simulink model "Smart_City_QCar2_self_driving_stack"  (R2024b)
settings: Solver=ode1  StartTime=0.0  StopTime=inf  FixedStep=Controller_Sample_Time  RelTol=1e-3  EnableMultiTasking=on
values from neighbouring files (symbols this model uses):
  angles_qcar2 = angles_new_qcar2(2: length (angles_new_qcar2), width (angles_new_qcar2)-5)    [Setup_QCar1and2_params.m]
  Audio_Sample_Time = 0.3    [Setup_QCar1and2_params.m]
  cal_pos = [0, 0, 0]    [Setup_QCar1and2_params.m]
  cameraStepSize = 3e-2    (= 0.03)    [Setup_QCar1and2_params.m]
  Cobra_Start = [0 0 0 0 0 0 0 0 0 0 0 0 ... (192000 elements, 192000x1)]    [QCar_Sounds.mat]
  Controller_Sample_Time = CSI_Sample_Time/10    (= 0.00166666666667)    [Setup_QCar1and2_params.m]
  CSI_Sample_Time = 1/60    (= 0.0166666666667)    [Setup_QCar1and2_params.m]
  engine = [0.455749511719 0.619506835938 0.612854003906 0.499603271484 0.347473144531 0.278045654297 0.304656982422 0.258544921875 0.100128173828 0.0902099609375 0.341461181641 0.515716552734 ... (88200 elements, 44100x2)]    [QCar_Sounds.mat]
  GyroKF_P0 = eye(2)    [Setup_QCar1and2_params.m]
  GyroKF_Q = diag([0.01, 0.001])    [Setup_QCar1and2_params.m]
  GyroKF_R = 0.01    [Setup_QCar1and2_params.m]
  GyroKF_X0 = [0;0]    [Setup_QCar1and2_params.m]
  honk = [0.01708984375 0.0179443359375 0.018798828125 0.019775390625 0.0209655761719 0.0218505859375 0.0221557617188 0.0223693847656 0.022705078125 0.023681640625 0.0252075195312 0.0257263183594 ... (43568 elements, 21784x2)]    [QCar_Sounds.mat]
  ImageDisplay_Sample_Time = CSI_Sample_Time*6    (= 0.1)    [Setup_QCar1and2_params.m]
  Initialization_Time = 5    [Setup_QCar1and2_params.m]
  LiDAR_Sample_Time = CSI_Sample_Time*3    (= 0.05)    [Setup_QCar1and2_params.m]
  map_mask = [1 1 1 0 0 1 0]    [Setup_QCar1and2_params.m]
  NN_Sample_Time = RealSense_Sample_Time*1    (= 0.0333333333333)    [Setup_QCar1and2_params.m]
  path_x = [0.826 0.836 0.846 0.856 0.866 0.876 0.886 0.896 0.906 0.916 0.926 0.936 ... (740 elements, 740x1)]    [SDCS_Paths_7.mat]
  path_x2 = [-0.614 -0.604 -0.594 -0.584 -0.574 -0.564 -0.554 -0.544 -0.534 -0.524 -0.514 -0.504 ... (1090 elements, 1090x1)]    [SDCS_Paths_7.mat]
  path_x3 = [-0.614 -0.603821428571 -0.593642857143 -0.583464285714 -0.573285714286 -0.563107142857 -0.552928571429 -0.54275 -0.532571428571 -0.522392857143 -0.512214285714 -0.502035714286 ... (714 elements, 714x1)]    [SDCS_Paths_7.mat]
  path_x4 = [-0.614 -0.604 -0.594 -0.584 -0.574 -0.564 -0.554 -0.544 -0.534 -0.524 -0.514 -0.504 ... (1761 elements, 1761x1)]    [SDCS_Paths_7.mat]
  path_x5 = [1.436 1.42588571429 1.41577142857 1.40565714286 1.39554285714 1.38542857143 1.37531428571 1.3652 1.35508571429 1.34497142857 1.33485714286 1.32474285714 ... (574 elements, 574x1)]    [SDCS_Paths_7.mat]
  path_x6 = [1.436 1.42588571429 1.41577142857 1.40565714286 1.39554285714 1.38542857143 1.37531428571 1.3652 1.35508571429 1.34497142857 1.33485714286 1.32474285714 ... (1288 elements, 1288x1)]    [SDCS_Paths_7.mat]
  path_x7 = [-1.5778487585 -1.56959877056 -1.56127865467 -1.55288878259 -1.54442952915 -1.53590127231 -1.52730439309 -1.51863927561 -1.50990630701 -1.50110587746 -1.49223838016 -1.4833042113 ... (2260 elements, 2260x1)]    [SDCS_Paths_7.mat]
  path_y = [-1.0887 -1.0887 -1.0887 -1.0887 -1.0887 -1.0887 -1.0887 -1.0887 -1.0887 -1.0887 -1.0887 -1.0887 ... (740 elements, 740x1)]    [SDCS_Paths_7.mat]
  path_y2 = [-1.0887 -1.0887 -1.0887 -1.0887 -1.0887 -1.0887 -1.0887 -1.0887 -1.0887 -1.0887 -1.0887 -1.0887 ... (1090 elements, 1090x1)]    [SDCS_Paths_7.mat]
  path_y3 = [-1.0887 -1.0887 -1.0887 -1.0887 -1.0887 -1.0887 -1.0887 -1.0887 -1.0887 -1.0887 -1.0887 -1.0887 ... (714 elements, 714x1)]    [SDCS_Paths_7.mat]
  path_y4 = [-1.0887 -1.0887 -1.0887 -1.0887 -1.0887 -1.0887 -1.0887 -1.0887 -1.0887 -1.0887 -1.0887 -1.0887 ... (1761 elements, 1761x1)]    [SDCS_Paths_7.mat]
  path_y5 = [-0.8157 -0.8157 -0.8157 -0.8157 -0.8157 -0.8157 -0.8157 -0.8157 -0.8157 -0.8157 -0.8157 -0.8157 ... (574 elements, 574x1)]    [SDCS_Paths_7.mat]
  path_y6 = [-0.8157 -0.8157 -0.8157 -0.8157 -0.8157 -0.8157 -0.8157 -0.8157 -0.8157 -0.8157 -0.8157 -0.8157 ... (1288 elements, 1288x1)]    [SDCS_Paths_7.mat]
  path_y7 = [-0.614490295955 -0.61974988896 -0.624981792226 -0.630185771997 -0.635361595765 -0.640509032279 -0.645627851559 -0.6507178249 -0.655778724888 -0.660810325409 -0.665812401655 -0.670784730139 ... (2260 elements, 2260x1)]    [SDCS_Paths_7.mat]
  put_me_down = [0 0 0 0 0 0 0 0 0 0 0 0 ... (335870 elements, 167935x2)]    [QCar_Sounds.mat]
  qcar2_lidar_to_map_rotation = 0    [Setup_QCar1and2_params.m]
  QCarEKF_L = 0.24    [Setup_QCar1and2_params.m]
  QCarEKF_P0 = eye(3)    [Setup_QCar1and2_params.m]
  QCarEKF_Q = diag([0.00001, 0.00001, 0.00001])    [Setup_QCar1and2_params.m]
  QCarEKF_R_combined = diag([0.1, 0.1, 0.01])    [Setup_QCar1and2_params.m]
  QCarEKF_R_heading = diag(0.1)    [Setup_QCar1and2_params.m]
  QcarKF_X0 = [0; 0; 0]    [Setup_QCar1and2_params.m]
  range_qcar2 = distance_new_qcar2(2: length (distance_new_qcar2), width (distance_new_qcar2)-5)    [Setup_QCar1and2_params.m]
  RealSense_Sample_Time = CSI_Sample_Time*2    (= 0.0333333333333)    [Setup_QCar1and2_params.m]
  truck_start = [0.00137329101562 0.00115966796875 0.0006103515625 0.000762939453125 0.00115966796875 0.00198364257812 0.00115966796875 0.000762939453125 0.00137329101562 0.00115966796875 0.00115966796875 0.000762939453125 ... (60000 elements, 60000x1)]    [QCar_Sounds.mat]
undefined symbols (not defined in the file or in its folder): DiscIntNeverNeededParam, gcbh, height, HIL, Joystick_Sample_Time, JPEG, left, Point, qc_get_step_size, top, video_display_show, width
libraries: quarc_library x65, simulink_extras x12, simulink x8
(part 4 of 5)

== system Smart_City_QCar2_self_driving_stack/QCar 2/QCar Control/QCar I//O/Audio ==
  Honk : Inport
  Arm : Inport  Port=2
  put_me_down : Inport  Port=3
  Volume : Inport  Port=4
  Car Horn1 : Constant  Value=[honk; honk]  VectorParams1D=off  OutDataTypeStr=single  SampleTime=Audio_Sample_Time
  Car Speaker1 : Subsystem
  Data Type Conversion : DataTypeConversion  OutDataTypeStr=single  SaturateOnIntegerOverflow=off  RndMeth=Floor
  From3 : From  Commented=on  GotoTag=Volume
  Old Car Engine2 : Constant  Commented=on  Value=engine  VectorParams1D=off  OutDataTypeStr=single  SampleTime=Audio_Sample_Time
  Old Car Engine3 : Constant  Commented=on  Value=truck_start  VectorParams1D=off  OutDataTypeStr=single  SampleTime=1
  Old Car Engine4 : Constant  Value=Cobra_Start  VectorParams1D=off  OutDataTypeStr=single  SampleTime=Audio_Sample_Time
  Old Car Engine5 : Constant  Value=put_me_down  VectorParams1D=off  OutDataTypeStr=single  SampleTime=Audio_Sample_Time
  Product11 : Product
  Product5 : Product
  Product8 : Product  Commented=on
  Rate Transition{,1,4..5} (4 alike) : RateTransition
  Rate Transition3 : RateTransition  Commented=on
  Subsystem2 : Subsystem  Commented=on
  Subsystem3 : Subsystem  Commented=on
  Subsystem4 : Subsystem
  Subsystem5 : Subsystem
  Volume4 : Gain  Commented=on  Gain=1/30  ParamDataTypeStr=double  OutDataTypeStr=single
  Volume5 : Gain  Gain=5/30  ParamDataTypeStr=double  OutDataTypeStr=single
  Volume7 : Gain  Commented=on  Gain=30/30  ParamDataTypeStr=double  OutDataTypeStr=single
  Volume8 : Gain  Gain=30/30*1  ParamDataTypeStr=double  OutDataTypeStr=single
  Volume9 : Gain  Gain=20/30  ParamDataTypeStr=double  OutDataTypeStr=single
  wires:
  Honk/1 -> Rate Transition/1
  Arm/1 -> Rate Transition1/1
  Rate Transition1/1 -> Subsystem2/Enable, Product5/2, Subsystem4/Trigger
  Old Car Engine2/1 -> Volume4/1
  Rate Transition/1 -> Product5/1
  Car Horn1/1 -> Volume5/1
  Old Car Engine3/1 -> Volume7/1
  Volume7/1 -> Subsystem3/1(In1)
  Product5/1 -> Car Speaker1/Enable
  Old Car Engine5/1 -> Volume9/1
  Volume9/1 -> Subsystem5/1(In1)
  Rate Transition4/1 -> Subsystem5/Enable
  put_me_down/1 -> Rate Transition4/1
  Volume/1 -> Rate Transition5/1
  Rate Transition5/1 -> Data Type Conversion/1
  From3/1 -> Product8/1
  Product8/1 -> Subsystem2/1(In1)
  Volume4/1 -> Product8/2
  [Volume] -> Product11/1
  Product11/1 -> Car Speaker1/1(chs)
  Volume5/1 -> Product11/2
  Data Type Conversion/1 -> [Volume]
  Old Car Engine4/1 -> Volume8/1
  Volume8/1 -> Subsystem4/1(In1)

== system Smart_City_QCar2_self_driving_stack/QCar 2/QCar Control/QCar I//O/Greater Than Threshold ==
  Signal : Inport
  Threshold : Inport  Port=2
  Duration : Inport  Port=3
  Data Type Conversion : DataTypeConversion  SaturateOnIntegerOverflow=off  RndMeth=Floor
  Discrete-Time Integrator : DiscreteIntegrator  Priority=1  ExternalReset=level  SampleTime=qc_get_step_size  ICPrevOutput=DiscIntNeverNeededParam  ICPrevScaledInput=DiscIntNeverNeededParam
  Logical Operator : Logic  Operator=NOT  AllPortsSameDT=off  OutDataTypeStr=boolean
  Relational Operator : RelationalOperator  InputSameDT=off
  Relational Operator1 : RelationalOperator  InputSameDT=off
  elapsed : Outport  VectorParamsAs1DForOutWhenUnconnected=off
  time : Outport  Port=2  VectorParamsAs1DForOutWhenUnconnected=off
  wires:
  Relational Operator1/1 -> elapsed/1
  Duration/1 -> Relational Operator1/2
  Discrete-Time Integrator/1 -> time/1, Relational Operator1/1
  Logical Operator/1 -> Discrete-Time Integrator/2
  Relational Operator/1 -> Logical Operator/1, Data Type Conversion/1
  Threshold/1 -> Relational Operator/2
  Signal/1 -> Relational Operator/1
  Data Type Conversion/1 -> Discrete-Time Integrator/1

== system Smart_City_QCar2_self_driving_stack/QCar 2/QCar Control/QCar I//O/LEDs ==
  note: Headlights, Brakes, Left, Right
  Throttle : Inport
  Steering : Inport  Port=2
  Speed : Inport  Port=3
  Hazzard : Inport  Port=4
  AND : Logic  IconShape=distinctive  AllPortsSameDT=off  OutDataTypeStr=boolean
  Constant : Constant  OutDataTypeStr=boolean
  Constant1 : Constant  Value=10
  Constant{2,4,6..7} (4 alike) : Constant  Value=.1
  Constant3 : Constant  Value=0
  Constant5 : Constant  Value=0
  Constant8 : Constant  Value=eps
  Demux : Demux
  Gain : Gain  Gain=-1
  Gain1 : Gain  Gain=-1
  Greater Than Threshold : Subsystem
  Greater Than Threshold1 : Subsystem
  Less Than Threshold : Subsystem
  Less Than Threshold1 : Subsystem
  Less Than Threshold2 : Subsystem
  Less Than Threshold3 : Subsystem
  Mux : Mux
  OR : Logic  Operator=OR  IconShape=distinctive  AllPortsSameDT=off  OutDataTypeStr=boolean
  Radians to Degrees : simulink_extras/Transformations/Radians to Degrees
  indicatorAndLamps : Subsystem
  LEDs : Outport
  wires:
  indicatorAndLamps/1(LEDs) -> LEDs/1
  Steering/1 -> Radians to Degrees/1
  Radians to Degrees/1 -> Less Than Threshold/1(Signal), Greater Than Threshold/1(Signal)
  Constant1/1 -> Gain/1, Greater Than Threshold/2(Threshold)
  Constant2/1 -> Less Than Threshold/3(Duration), Greater Than Threshold/3(Duration)
  Greater Than Threshold/1(elapsed) -> Mux/3
  Gain/1 -> Less Than Threshold/2(Threshold)
  Less Than Threshold/1(elapsed) -> Mux/4
  Speed/1 -> Less Than Threshold3/1(Signal), Greater Than Threshold1/1(Signal), Less Than Threshold1/1(Signal)
  Constant3/1 -> Less Than Threshold1/2(Threshold)
  Constant4/1 -> Less Than Threshold1/3(Duration)
  Less Than Threshold1/1(elapsed) -> indicatorAndLamps/5(reverse)
  Throttle/1 -> Less Than Threshold2/1(Signal)
  Constant5/1 -> Less Than Threshold2/2(Threshold)
  Constant6/1 -> Less Than Threshold2/3(Duration)
  Hazzard/1 -> indicatorAndLamps/6(hazard)
  Less Than Threshold2/1(elapsed) -> OR/1
  Constant7/1 -> Less Than Threshold3/3(Duration), Greater Than Threshold1/3(Duration)
  Constant8/1 -> Gain1/1, Less Than Threshold3/2(Threshold)
  Less Than Threshold3/1(elapsed) -> AND/1
  Greater Than Threshold1/1(elapsed) -> AND/2
  AND/1 -> OR/2
  Gain1/1 -> Greater Than Threshold1/2(Threshold)
  Constant/1 -> Mux/1
  OR/1 -> Mux/2
  Demux/3 -> indicatorAndLamps/3(Indicate Left)
  Demux/2 -> indicatorAndLamps/2(brakes)
  Demux/4 -> indicatorAndLamps/4(Indicate Right)
  Demux/1 -> indicatorAndLamps/1(headlamps)
  Mux/1 -> Demux/1

== system Smart_City_QCar2_self_driving_stack/QCar 2/QCar Control/QCar I//O/Less Than Threshold1 ==
  Signal : Inport
  Threshold : Inport  Port=2
  Duration : Inport  Port=3
  Data Type Conversion : DataTypeConversion  SaturateOnIntegerOverflow=off  RndMeth=Floor
  Discrete-Time Integrator : DiscreteIntegrator  Priority=1  ExternalReset=level  SampleTime=qc_get_step_size  ICPrevOutput=DiscIntNeverNeededParam  ICPrevScaledInput=DiscIntNeverNeededParam
  Logical Operator : Logic  Operator=NOT  AllPortsSameDT=off  OutDataTypeStr=boolean
  Relational Operator : RelationalOperator  Operator=<  InputSameDT=off
  Relational Operator1 : RelationalOperator  InputSameDT=off
  elapsed : Outport  VectorParamsAs1DForOutWhenUnconnected=off
  time : Outport  Port=2  VectorParamsAs1DForOutWhenUnconnected=off
  wires:
  Data Type Conversion/1 -> Discrete-Time Integrator/1
  Signal/1 -> Relational Operator/1
  Threshold/1 -> Relational Operator/2
  Relational Operator/1 -> Data Type Conversion/1, Logical Operator/1
  Logical Operator/1 -> Discrete-Time Integrator/2
  Discrete-Time Integrator/1 -> Relational Operator1/1, time/1
  Duration/1 -> Relational Operator1/2
  Relational Operator1/1 -> elapsed/1

== system Smart_City_QCar2_self_driving_stack/QCar 2/QCar Control/QCar I//O/basicSpeedEstimation ==
  note: speedEstimation Module:
      |
      | This subsystem converts the motor speed measurements in counts/s to a useful longitudinal car speed in m/s.
      |
      | Inputs:
      | motorSpeed (counts/s) n/a : Drive motor speed measured using an encoder
      |
      | Outputs:
      | longitudinalCarSpeed (m/s) n/a : The platform's longitudinal speed (along the front-rear axis direction)
  note: (Diff. pinion*pinion)/(Spur*Diff. spur)
  note: v = 2*pi*r * omega (if omega is in rot/s)
      | v = r * omega (if omega is in rad/s)
      | r = 0.0342 m
  note: Estimate car speed from motor encoder counts rate
  motorSpeed (counts/s) : Inport
  counts to rotations : Gain  Gain=1/720/4
  gear ratios : Gain  Gain=(13*19)/(70*37)
  rot/s to rad/s : Gain  Gain=2*pi
  wheel radius : Gain  Gain=0.0342
  longitudinalCarSpeed (m/s) : Outport  VectorParamsAs1DForOutWhenUnconnected=off
  wires:
  gear ratios/1 -> rot/s to rad/s/1  "shaft speed (rots/s)"
  wheel radius/1 -> longitudinalCarSpeed (m/s)/1  "wheel speed (m/s)"
  counts to rotations/1 -> gear ratios/1  "motor speed (rot/s)"
  rot/s to rad/s/1 -> wheel radius/1  "wheel speed (rad/s)"
  motorSpeed (counts/s)/1 -> counts to rotations/1

== system Smart_City_QCar2_self_driving_stack/QCar 2/QCar Control/QCar I//O/basicSpeedEstimation1 ==
  note: Estimate car speed from motor encoder counts rate
  note: v = 2*pi*r * omega (if omega is in rot/s)
      | v = r * omega (if omega is in rad/s)
      | r = 0.0342 m
  note: (Diff. pinion*pinion)/(Spur*Diff. spur)
  note: speedEstimation Module:
      |
      | This subsystem converts the motor speed measurements in counts/s to a useful longitudinal car speed in m/s.
      |
      | Inputs:
      | motorSpeed (counts/s) n/a : Drive motor speed measured using an encoder
      |
      | Outputs:
      | longitudinalCarSpeed (m/s) n/a : The platform's longitudinal speed (along the front-rear axis direction)
  motorSpeed (counts/s) : Inport
  counts to rotations : Gain  Gain=1/720/4
  gear ratios : Gain  Gain=(13*19)/(70*37)
  rot/s to rad/s : Gain  Gain=2*pi
  wheel radius : Gain  Gain=0.0342
  longitudinalCarSpeed (m/s) : Outport  VectorParamsAs1DForOutWhenUnconnected=off
  wires:
  motorSpeed (counts/s)/1 -> counts to rotations/1
  rot/s to rad/s/1 -> wheel radius/1  "wheel speed (rad/s)"
  counts to rotations/1 -> gear ratios/1  "motor speed (rot/s)"
  wheel radius/1 -> longitudinalCarSpeed (m/s)/1  "wheel speed (m/s)"
  gear ratios/1 -> rot/s to rad/s/1  "shaft speed (rots/s)"

== system Smart_City_QCar2_self_driving_stack/QCar 2/QCar Control/QCar I//O/Audio/Car Speaker1 ==
  chs : Inport
  Enable : EnablePort
  Audio Play : quarc_library/Multimedia/Audio Play  device_id=demixer  sample_rate=44100  num_channels=[]  buffer_size=44100  sample_time=-1
      settings: SourceProductName=QUARC Targets
  wires:
  chs/1 -> Audio Play/1

== system Smart_City_QCar2_self_driving_stack/QCar 2/QCar Control/QCar I//O/Audio/Subsystem2 ==
  In1 : Inport
  Enable : EnablePort
  Audio Play : quarc_library/Multimedia/Audio Play  device_id=demixer  sample_rate=41000  num_channels=[]  buffer_size=length (engine)  sample_time=-1
      settings: SourceProductName=QUARC Targets
  wires:
  In1/1 -> Audio Play/1

== system Smart_City_QCar2_self_driving_stack/QCar 2/QCar Control/QCar I//O/Audio/Subsystem3 ==
  In1 : Inport
  Enable : EnablePort
  Audio Play : quarc_library/Multimedia/Audio Play  device_id=demixer  sample_rate=48000  num_channels=[]  buffer_size=length(truck_start)  sample_time=-1
      settings: SourceProductName=QUARC Targets
  wires:
  In1/1 -> Audio Play/1

== system Smart_City_QCar2_self_driving_stack/QCar 2/QCar Control/QCar I//O/Audio/Subsystem4 ==
  In1 : Inport
  Trigger : TriggerPort  VariantControl=Variant  PortDimensions=1
  Audio Play : quarc_library/Multimedia/Audio Play  device_id=demixer  sample_rate=48000  num_channels=[]  buffer_size=length(Cobra_Start)  sample_time=-1
      settings: SourceProductName=QUARC Targets
  wires:
  In1/1 -> Audio Play/1

== system Smart_City_QCar2_self_driving_stack/QCar 2/QCar Control/QCar I//O/Audio/Subsystem5 ==
  In1 : Inport
  Enable : EnablePort
  Audio Play : quarc_library/Multimedia/Audio Play  device_id=demixer  sample_rate=48000  num_channels=[]  buffer_size=length(put_me_down)  sample_time=-1
      settings: SourceProductName=QUARC Targets
  wires:
  In1/1 -> Audio Play/1

== system Smart_City_QCar2_self_driving_stack/QCar 2/QCar Control/QCar I//O/LEDs/Greater Than Threshold ==
  Signal : Inport
  Threshold : Inport  Port=2
  Duration : Inport  Port=3
  Data Type Conversion : DataTypeConversion  SaturateOnIntegerOverflow=off  RndMeth=Floor
  Discrete-Time Integrator : DiscreteIntegrator  Priority=1  ExternalReset=level  SampleTime=qc_get_step_size  ICPrevOutput=DiscIntNeverNeededParam  ICPrevScaledInput=DiscIntNeverNeededParam
  Logical Operator : Logic  Operator=NOT  AllPortsSameDT=off  OutDataTypeStr=boolean
  Relational Operator : RelationalOperator  InputSameDT=off
  Relational Operator1 : RelationalOperator  InputSameDT=off
  elapsed : Outport  VectorParamsAs1DForOutWhenUnconnected=off
  time : Outport  Port=2  VectorParamsAs1DForOutWhenUnconnected=off
  wires:
  Relational Operator1/1 -> elapsed/1
  Duration/1 -> Relational Operator1/2
  Discrete-Time Integrator/1 -> time/1, Relational Operator1/1
  Logical Operator/1 -> Discrete-Time Integrator/2
  Relational Operator/1 -> Logical Operator/1, Data Type Conversion/1
  Threshold/1 -> Relational Operator/2
  Signal/1 -> Relational Operator/1
  Data Type Conversion/1 -> Discrete-Time Integrator/1

== system Smart_City_QCar2_self_driving_stack/QCar 2/QCar Control/QCar I//O/LEDs/Greater Than Threshold1 ==
  Signal : Inport
  Threshold : Inport  Port=2
  Duration : Inport  Port=3
  Data Type Conversion : DataTypeConversion  SaturateOnIntegerOverflow=off  RndMeth=Floor
  Discrete-Time Integrator : DiscreteIntegrator  Priority=1  ExternalReset=level  SampleTime=qc_get_step_size  ICPrevOutput=DiscIntNeverNeededParam  ICPrevScaledInput=DiscIntNeverNeededParam
  Logical Operator : Logic  Operator=NOT  AllPortsSameDT=off  OutDataTypeStr=boolean
  Relational Operator : RelationalOperator  InputSameDT=off
  Relational Operator1 : RelationalOperator  InputSameDT=off
  elapsed : Outport  VectorParamsAs1DForOutWhenUnconnected=off
  time : Outport  Port=2  VectorParamsAs1DForOutWhenUnconnected=off
  wires:
  Relational Operator1/1 -> elapsed/1
  Duration/1 -> Relational Operator1/2
  Discrete-Time Integrator/1 -> time/1, Relational Operator1/1
  Logical Operator/1 -> Discrete-Time Integrator/2
  Relational Operator/1 -> Logical Operator/1, Data Type Conversion/1
  Threshold/1 -> Relational Operator/2
  Signal/1 -> Relational Operator/1
  Data Type Conversion/1 -> Discrete-Time Integrator/1

== system Smart_City_QCar2_self_driving_stack/QCar 2/QCar Control/QCar I//O/LEDs/Less Than Threshold ==
  Signal : Inport
  Threshold : Inport  Port=2
  Duration : Inport  Port=3
  Data Type Conversion : DataTypeConversion  SaturateOnIntegerOverflow=off  RndMeth=Floor
  Discrete-Time Integrator : DiscreteIntegrator  Priority=1  ExternalReset=level  SampleTime=qc_get_step_size  ICPrevOutput=DiscIntNeverNeededParam  ICPrevScaledInput=DiscIntNeverNeededParam
  Logical Operator : Logic  Operator=NOT  AllPortsSameDT=off  OutDataTypeStr=boolean
  Relational Operator : RelationalOperator  Operator=<  InputSameDT=off
  Relational Operator1 : RelationalOperator  InputSameDT=off
  elapsed : Outport  VectorParamsAs1DForOutWhenUnconnected=off
  time : Outport  Port=2  VectorParamsAs1DForOutWhenUnconnected=off
  wires:
  Relational Operator1/1 -> elapsed/1
  Duration/1 -> Relational Operator1/2
  Discrete-Time Integrator/1 -> time/1, Relational Operator1/1
  Logical Operator/1 -> Discrete-Time Integrator/2
  Relational Operator/1 -> Logical Operator/1, Data Type Conversion/1
  Threshold/1 -> Relational Operator/2
  Signal/1 -> Relational Operator/1
  Data Type Conversion/1 -> Discrete-Time Integrator/1

== system Smart_City_QCar2_self_driving_stack/QCar 2/QCar Control/QCar I//O/LEDs/Less Than Threshold1 ==
  Signal : Inport
  Threshold : Inport  Port=2
  Duration : Inport  Port=3
  Data Type Conversion : DataTypeConversion  SaturateOnIntegerOverflow=off  RndMeth=Floor
  Discrete-Time Integrator : DiscreteIntegrator  Priority=1  ExternalReset=level  SampleTime=qc_get_step_size  ICPrevOutput=DiscIntNeverNeededParam  ICPrevScaledInput=DiscIntNeverNeededParam
  Logical Operator : Logic  Operator=NOT  AllPortsSameDT=off  OutDataTypeStr=boolean
  Relational Operator : RelationalOperator  Operator=<  InputSameDT=off
  Relational Operator1 : RelationalOperator  InputSameDT=off
  elapsed : Outport  VectorParamsAs1DForOutWhenUnconnected=off
  time : Outport  Port=2  VectorParamsAs1DForOutWhenUnconnected=off
  wires:
  Data Type Conversion/1 -> Discrete-Time Integrator/1
  Signal/1 -> Relational Operator/1
  Threshold/1 -> Relational Operator/2
  Relational Operator/1 -> Data Type Conversion/1, Logical Operator/1
  Logical Operator/1 -> Discrete-Time Integrator/2
  Discrete-Time Integrator/1 -> Relational Operator1/1, time/1
  Duration/1 -> Relational Operator1/2
  Relational Operator1/1 -> elapsed/1

== system Smart_City_QCar2_self_driving_stack/QCar 2/QCar Control/QCar I//O/LEDs/Less Than Threshold2 ==
  Signal : Inport
  Threshold : Inport  Port=2
  Duration : Inport  Port=3
  Data Type Conversion : DataTypeConversion  SaturateOnIntegerOverflow=off  RndMeth=Floor
  Discrete-Time Integrator : DiscreteIntegrator  Priority=1  ExternalReset=level  SampleTime=qc_get_step_size  ICPrevOutput=DiscIntNeverNeededParam  ICPrevScaledInput=DiscIntNeverNeededParam
  Logical Operator : Logic  Operator=NOT  AllPortsSameDT=off  OutDataTypeStr=boolean
  Relational Operator : RelationalOperator  Operator=<  InputSameDT=off
  Relational Operator1 : RelationalOperator  InputSameDT=off
  elapsed : Outport  VectorParamsAs1DForOutWhenUnconnected=off
  time : Outport  Port=2  VectorParamsAs1DForOutWhenUnconnected=off
  wires:
  Relational Operator1/1 -> elapsed/1
  Duration/1 -> Relational Operator1/2
  Discrete-Time Integrator/1 -> time/1, Relational Operator1/1
  Logical Operator/1 -> Discrete-Time Integrator/2
  Relational Operator/1 -> Logical Operator/1, Data Type Conversion/1
  Threshold/1 -> Relational Operator/2
  Signal/1 -> Relational Operator/1
  Data Type Conversion/1 -> Discrete-Time Integrator/1

== system Smart_City_QCar2_self_driving_stack/QCar 2/QCar Control/QCar I//O/LEDs/Less Than Threshold3 ==
  Signal : Inport
  Threshold : Inport  Port=2
  Duration : Inport  Port=3
  Data Type Conversion : DataTypeConversion  SaturateOnIntegerOverflow=off  RndMeth=Floor
  Discrete-Time Integrator : DiscreteIntegrator  Priority=1  ExternalReset=level  SampleTime=qc_get_step_size  ICPrevOutput=DiscIntNeverNeededParam  ICPrevScaledInput=DiscIntNeverNeededParam
  Logical Operator : Logic  Operator=NOT  AllPortsSameDT=off  OutDataTypeStr=boolean
  Relational Operator : RelationalOperator  Operator=<  InputSameDT=off
  Relational Operator1 : RelationalOperator  InputSameDT=off
  elapsed : Outport  VectorParamsAs1DForOutWhenUnconnected=off
  time : Outport  Port=2  VectorParamsAs1DForOutWhenUnconnected=off
  wires:
  Data Type Conversion/1 -> Discrete-Time Integrator/1
  Signal/1 -> Relational Operator/1
  Threshold/1 -> Relational Operator/2
  Relational Operator/1 -> Data Type Conversion/1, Logical Operator/1
  Logical Operator/1 -> Discrete-Time Integrator/2
  Discrete-Time Integrator/1 -> Relational Operator1/1, time/1
  Duration/1 -> Relational Operator1/2
  Relational Operator1/1 -> elapsed/1

== system Smart_City_QCar2_self_driving_stack/QCar 2/QCar Control/QCar I//O/LEDs/indicatorAndLamps ==
  note: Turn Indicators:
      | # Longditudal Lateral Color
      | 1 Rear Left Amber
      | 2 Rear Right Amber
      | 3 Front Left Amber
      | 4 Front Right Amber
      |
      | Lamps:
      | # Longditudal Lateral Color
      | 5 Rear Left Red
      | 6 Rear Right Red
      | 7 Front Left White
      | 8 Front Right White
  headlamps : Inport
  brakes : Inport  Port=2
  Indicate Left : Inport  Port=3
  Indicate Right : Inport  Port=4
  reverse : Inport  Port=5
  hazard : Inport  Port=6
  AND1 : Logic  IconShape=distinctive  AllPortsSameDT=off  OutDataTypeStr=boolean
  AND2 : Logic  Operator=OR  IconShape=distinctive  AllPortsSameDT=off  OutDataTypeStr=boolean
  AND3 : Logic  IconShape=distinctive  AllPortsSameDT=off  OutDataTypeStr=boolean
  AND4 : Logic  Operator=OR  IconShape=distinctive  AllPortsSameDT=off  OutDataTypeStr=boolean
  Data Type Conversion : DataTypeConversion  SaturateOnIntegerOverflow=off  RndMeth=Floor
  Data Type Conversion1 : DataTypeConversion  SaturateOnIntegerOverflow=off  RndMeth=Floor
  Light Off : Constant  Value=zeros(1,4)  OutDataTypeStr=boolean
  Light Off1 : Constant  Value=zeros(1,2)  OutDataTypeStr=boolean
  Light Off2 : Constant  Value=zeros(1,3)  OutDataTypeStr=boolean
  Mux : Mux  Inputs=8
  Pulsing Light : DiscretePulseGenerator  Period=1/qc_get_step_size  PulseWidth=1/2/qc_get_step_size  SampleTime=qc_get_step_size
  Steady Light : Constant  Value=ones(1,4)  OutDataTypeStr=boolean
  Steady Light1 : Constant  Value=ones(1,2)  OutDataTypeStr=boolean
  Steady Light2 : Constant  Value=ones(1,3)  OutDataTypeStr=boolean
  Switch1 : Switch  Criteria=u2 > Threshold  SaturateOnIntegerOverflow=off  InputSameDT=off
  Switch2 : Switch  Criteria=u2 > Threshold  SaturateOnIntegerOverflow=off  InputSameDT=off
  Switch3 : Switch  Criteria=u2 > Threshold  SaturateOnIntegerOverflow=off  InputSameDT=off
  LEDs : Outport  VectorParamsAs1DForOutWhenUnconnected=off
  wires:
  Light Off/1 -> Switch2/3
  Steady Light/1 -> Switch2/1
  Indicate Right/1 -> AND4/2
  Mux/1 -> Data Type Conversion1/1
  Pulsing Light/1 -> Data Type Conversion/1
  Data Type Conversion/1 -> AND3/2, AND1/2
  Data Type Conversion1/1 -> LEDs/1
  Indicate Left/1 -> AND2/2
  Switch2/1 -> Mux/5
  AND3/1 -> Mux/3, Mux/1
  AND1/1 -> Mux/4, Mux/2
  Switch1/1 -> Mux/6
  Switch3/1 -> Mux/7, Mux/8
  brakes/1 -> Switch2/2
  reverse/1 -> Switch1/2
  headlamps/1 -> Switch3/2
  hazard/1 -> AND2/1, AND4/1
  AND2/1 -> AND3/1
  AND4/1 -> AND1/1
  Light Off1/1 -> Switch1/3
  Light Off2/1 -> Switch3/3
  Steady Light1/1 -> Switch1/1
  Steady Light2/1 -> Switch3/1

== matlab function Smart_City_QCar2_self_driving_stack/QCar 2/LiDAR/Match Scans/MATLAB Function ==
  data: new_range output size=SPR_qcar2 [..SPR_qcar2]; range input [1..SPR_qcar2]; angles input [1..SPR_qcar2]; new_angles output size=SPR_qcar2 [..SPR_qcar2]
function [new_range, new_angles]  = clean_zero_readings(range, angles)
range_indicies = find (range == 0);
range(range_indicies) = [];
angles(range_indicies) = [];
new_range = range;
new_angles = angles;
end

== matlab function Smart_City_QCar2_self_driving_stack/Speed & Steering Commander/Realsense Obstacle Detection Speed Adjust/MATLAB Function ==
  data: obstacle_distance input; speed_cmd output; stop_distance input; nominal_tracking_distance input; nominal_speed input
function speed_cmd = adaptive_cruise_control(obstacle_distance, stop_distance, nominal_tracking_distance, nominal_speed)

speed_cmd = nominal_speed;

if obstacle_distance < stop_distance
    speed_cmd = sat(nominal_speed,0,-1);
    
elseif obstacle_distance < nominal_tracking_distance
    speed_cmd = nominal_speed/(nominal_tracking_distance-stop_distance)*obstacle_distance...
        - nominal_speed/(nominal_tracking_distance-stop_distance)*stop_distance;
    
end

function output = sat (input, max,min)
if input > max
    output = max;
elseif input < min
    output = min;
else
    output = input;
end

== matlab function Smart_City_QCar2_self_driving_stack/Speed & Steering Commander/Steering Based on LiDAR/Steering Commander ==
  data: steering output; aoa input
function steering  = steering_command(aoa)
steering = aoa;
if aoa < -pi
    steering = aoa+2*pi;
elseif aoa > pi
    steering = aoa-2*pi;
else
    steering = aoa;
end
end

== matlab function Smart_City_QCar2_self_driving_stack/Speed & Steering Commander/Path Commander/Path 7  Look Ahead Generator/Windowed Closest Point Locator *Feedback the location1 ==
  data: x input; location output; y input; x_array input; y_array input; window input; global_search input; distance output; previous_location input
function [location,distance] = find_closest_window_point(x,y,x_array,y_array, window, global_search, previous_location)
distance = 1e6;
location = previous_location;
array_length = length (x_array);

if (global_search == 1)
    
    %Search the whole array (usually at startup)
    for i =1:array_length
        d = (x-x_array(i))^2 + (y-y_array(i))^2;
        if d < distance
            distance = d;
            location = i;
        end
    end
    
else
    
    if (location + window) > array_length
        %We need to wrap from the end
        % loop one - end of array:
        for i = (location-window):array_length
            d = (x-x_array(i))^2 + (y-y_array(i))^2;
            if d < distance
                distance = d;
                location = i;
            end
        end
        % loop two - start of array:
        for i = 1:(location+window-array_length)
            d = (x-x_array(i))^2 + (y-y_array(i))^2;
            if d < distance
                distance = d;
                location = i;
            end
        end
        
    elseif (location-window) < 1
        %We need to wrap from the beginning
        % loop one - end of array:
        for i = (array_length+location-window):array_length
            d = (x-x_array(i))^2 + (y-y_array(i))^2;
            if d < distance
                distance = d;
                location = i;
            end
        end
        % loop two - start of array:
        for i = 1:(location+window)
            d = (x-x_array(i))^2 + (y-y_array(i))^2;
            if d < distance
                distance = d;
                location = i;
            end
        end
        
    else
        %no need to wrap
        for i = (location-window):(location+window)
            d = (x-x_array(i))^2 + (y-y_array(i))^2;
            if d < distance
                distance = d;
                location = i;
            end
        end
    end
    
end
distance = sqrt(distance);
end

== matlab function Smart_City_QCar2_self_driving_stack/RealSense Camera/obstacleDetection Markham March 22/Draw Lines Module ==
  data: img_in input; img_out output; pts input; color input
function img_out = drawLines(img_in, pts, color)

% Draw lines connecting the points using the provided color

% Inputs:
% u         : Input RGB Image (size = m by n)
% pts       : p x-y pairs of points (px) where markers are to be drawn
% color     : 1x3 matrix of RGB color values for each marker

% Outputs:
% y         : Output RGB Image with the markers drawn in (size = m by n)

%% Initialization
if size(img_in, 3) == 3
    img_out = img_in;
elseif size(img_in, 3) == 1
    img_out = cat(3, img_in, img_in, img_in);
end

[p, ~] = size(pts); % determine the number of points

%% Draw the lines
    for i = 1:p-1
        % determine the max(rows_difference, col_difference) between two
        % points
        itr = max(abs(pts(i,1) - pts(i+1,1)), abs(pts(i,2) - pts(i+1,2)));
        
        % generate linear spaces of row and col values between the pts
        row_vec = round(linspace(pts(i,1), pts(i+1,1), itr));
        col_vec = round(linspace(pts(i,2), pts(i+1,2), itr));
        
        % iterate through the values and shade them right

        for j = 1:itr
            img_out(row_vec(j), col_vec(j),1) = color(1);
            img_out(row_vec(j), col_vec(j),2) = color(2);
            img_out(row_vec(j), col_vec(j),3) = color(3);
        end
    end
end

== matlab function Smart_City_QCar2_self_driving_stack/Speed & Steering Commander/Path Commander/Path 1  Look Ahead Generator/Windowed Closest Point Locator *Feedback the location1 ==
  data: x input; location output; y input; x_array input; y_array input; window input; global_search input; distance output; previous_location input
function [location,distance] = find_closest_window_point(x,y,x_array,y_array, window, global_search, previous_location)
distance = 1e6;
location = previous_location;
array_length = length (x_array);

if (global_search == 1)
    
    %Search the whole array (usually at startup)
    for i =1:array_length
        d = (x-x_array(i))^2 + (y-y_array(i))^2;
        if d < distance
            distance = d;
            location = i;
        end
    end
    
else
    
    if (location + window) > array_length
        %We need to wrap from the end
        % loop one - end of array:
        for i = (location-window):array_length
            d = (x-x_array(i))^2 + (y-y_array(i))^2;
            if d < distance
                distance = d;
                location = i;
            end
        end
        % loop two - start of array:
        for i = 1:(location+window-array_length)
            d = (x-x_array(i))^2 + (y-y_array(i))^2;
            if d < distance
                distance = d;
                location = i;
            end
        end
        
    elseif (location-window) < 1
        %We need to wrap from the beginning
        % loop one - end of array:
        for i = (array_length+location-window):array_length
            d = (x-x_array(i))^2 + (y-y_array(i))^2;
            if d < distance
                distance = d;
                location = i;
            end
        end
        % loop two - start of array:
        for i = 1:(location+window)
            d = (x-x_array(i))^2 + (y-y_array(i))^2;
            if d < distance
                distance = d;
                location = i;
            end
        end
        
    else
        %no need to wrap
        for i = (location-window):(location+window)
            d = (x-x_array(i))^2 + (y-y_array(i))^2;
            if d < distance
                distance = d;
                location = i;
            end
        end
    end
    
end
distance = sqrt(distance);
end

== matlab function Smart_City_QCar2_self_driving_stack/Speed & Steering Commander/Path Commander/Path 2  Look Ahead Generator/Windowed Closest Point Locator *Feedback the location1 ==
  data: x input; location output; y input; x_array input; y_array input; window input; global_search input; distance output; previous_location input
function [location,distance] = find_closest_window_point(x,y,x_array,y_array, window, global_search, previous_location)
distance = 1e6;
location = previous_location;
array_length = length (x_array);

if (global_search == 1)
    
    %Search the whole array (usually at startup)
    for i =1:array_length
        d = (x-x_array(i))^2 + (y-y_array(i))^2;
        if d < distance
            distance = d;
            location = i;
        end
    end
    
else
    
    if (location + window) > array_length
        %We need to wrap from the end
        % loop one - end of array:
        for i = (location-window):array_length
            d = (x-x_array(i))^2 + (y-y_array(i))^2;
            if d < distance
                distance = d;
                location = i;
            end
        end
        % loop two - start of array:
        for i = 1:(location+window-array_length)
            d = (x-x_array(i))^2 + (y-y_array(i))^2;
            if d < distance
                distance = d;
                location = i;
            end
        end
        
    elseif (location-window) < 1
        %We need to wrap from the beginning
        % loop one - end of array:
        for i = (array_length+location-window):array_length
            d = (x-x_array(i))^2 + (y-y_array(i))^2;
            if d < distance
                distance = d;
                location = i;
            end
        end
        % loop two - start of array:
        for i = 1:(location+window)
            d = (x-x_array(i))^2 + (y-y_array(i))^2;
            if d < distance
                distance = d;
                location = i;
            end
        end
        
    else
        %no need to wrap
        for i = (location-window):(location+window)
            d = (x-x_array(i))^2 + (y-y_array(i))^2;
            if d < distance
                distance = d;
                location = i;
            end
        end
    end
    
end
distance = sqrt(distance);
end

== matlab function Smart_City_QCar2_self_driving_stack/RealSense Camera/obstacleDetection Markham March 22/Steering based image subselector ==
  data: pts output; depth input; distance output; steering input; minDistance input; maxDistance input; width input; height input; vertCenter input; maxSteering input; reduction input; maxSteeringWidth input
function [pts, distance] = estimateDepthInRegion(depth, steering, minDistance, maxDistance, width, height, vertCenter, maxSteering, reduction, maxSteeringWidth)
% Input: 640 x 360
[ROW, COL] = size(depth);
mark = COL/2 - (steering*(COL/2 - width/2)/maxSteering);
applied_width = max(width - abs(steering/maxSteeringWidth)*reduction*width, 60);
left_w = max(mark+1-(applied_width/2), 0); % pick the left end, but never let it get negative
right_w = min(left_w + applied_width, COL); % pick the right end, but never past the image width
upper_h = max(ROW*vertCenter-height/2+1, 0); % pick the upper end, but never let it get negative
lower_h = min(ROW*vertCenter+height/2, ROW); % pick the lower end, but never let it go past the image height
depth(:,1:40) = maxDistance; %this is to remove artifacts in the camera's left section
region = double(depth(upper_h:lower_h, left_w:right_w)); 
pts = [upper_h, left_w; upper_h, right_w; lower_h, right_w; lower_h, left_w; upper_h, left_w];
u_flat = reshape(region, 1, []);

temp = maxDistance*ones(1, length(u_flat));

for i = 1:length(u_flat)
    if (u_flat(i) >= minDistance) && (u_flat(i) <= maxDistance)
        temp(i) = u_flat(i);
    end
end

% u_flat(u_flat < minDistance) = [];
% u_flat(u_flat > maxDistance) = [];
% distance = mean(mean(u_flat));
distance = min(temp(:));

== matlab function Smart_City_QCar2_self_driving_stack/Speed & Steering Commander/Path Commander/Path 4  Look Ahead Generator/Windowed Closest Point Locator *Feedback the location1 ==
  data: x input; location output; y input; x_array input; y_array input; window input; global_search input; distance output; previous_location input
function [location,distance] = find_closest_window_point(x,y,x_array,y_array, window, global_search, previous_location)
distance = 1e6;
location = previous_location;
array_length = length (x_array);

if (global_search == 1)
    
    %Search the whole array (usually at startup)
    for i =1:array_length
        d = (x-x_array(i))^2 + (y-y_array(i))^2;
        if d < distance
            distance = d;
            location = i;
        end
    end
    
else
    
    if (location + window) > array_length
        %We need to wrap from the end
        % loop one - end of array:
        for i = (location-window):array_length
            d = (x-x_array(i))^2 + (y-y_array(i))^2;
            if d < distance
                distance = d;
                location = i;
            end
        end
        % loop two - start of array:
        for i = 1:(location+window-array_length)
            d = (x-x_array(i))^2 + (y-y_array(i))^2;
            if d < distance
                distance = d;
                location = i;
            end
        end
        
    elseif (location-window) < 1
        %We need to wrap from the beginning
        % loop one - end of array:
        for i = (array_length+location-window):array_length
            d = (x-x_array(i))^2 + (y-y_array(i))^2;
            if d < distance
                distance = d;
                location = i;
            end
        end
        % loop two - start of array:
        for i = 1:(location+window)
            d = (x-x_array(i))^2 + (y-y_array(i))^2;
            if d < distance
                distance = d;
                location = i;
            end
        end
        
    else
        %no need to wrap
        for i = (location-window):(location+window)
            d = (x-x_array(i))^2 + (y-y_array(i))^2;
            if d < distance
                distance = d;
                location = i;
            end
        end
    end
    
end
distance = sqrt(distance);
end

== matlab function Smart_City_QCar2_self_driving_stack/Speed & Steering Commander/Path Commander/Path 5  Look Ahead Generator/Windowed Closest Point Locator *Feedback the location1 ==
  data: x input; location output; y input; x_array input; y_array input; window input; global_search input; distance output; previous_location input
function [location,distance] = find_closest_window_point(x,y,x_array,y_array, window, global_search, previous_location)
distance = 1e6;
location = previous_location;
array_length = length (x_array);

if (global_search == 1)
    
    %Search the whole array (usually at startup)
    for i =1:array_length
        d = (x-x_array(i))^2 + (y-y_array(i))^2;
        if d < distance
            distance = d;
            location = i;
        end
    end
    
else
    
    if (location + window) > array_length
        %We need to wrap from the end
        % loop one - end of array:
        for i = (location-window):array_length
            d = (x-x_array(i))^2 + (y-y_array(i))^2;
            if d < distance
                distance = d;
                location = i;
            end
        end
        % loop two - start of array:
        for i = 1:(location+window-array_length)
            d = (x-x_array(i))^2 + (y-y_array(i))^2;
            if d < distance
                distance = d;
                location = i;
            end
        end
        
    elseif (location-window) < 1
        %We need to wrap from the beginning
        % loop one - end of array:
        for i = (array_length+location-window):array_length
            d = (x-x_array(i))^2 + (y-y_array(i))^2;
            if d < distance
                distance = d;
                location = i;
            end
        end
        % loop two - start of array:
        for i = 1:(location+window)
            d = (x-x_array(i))^2 + (y-y_array(i))^2;
            if d < distance
                distance = d;
                location = i;
            end
        end
        
    else
        %no need to wrap
        for i = (location-window):(location+window)
            d = (x-x_array(i))^2 + (y-y_array(i))^2;
            if d < distance
                distance = d;
                location = i;
            end
        end
    end
    
end
distance = sqrt(distance);
end

== matlab function Smart_City_QCar2_self_driving_stack/Speed & Steering Commander/Path Commander/Path 6  Look Ahead Generator/Windowed Closest Point Locator *Feedback the location1 ==
  data: x input; location output; y input; x_array input; y_array input; window input; global_search input; distance output; previous_location input
function [location,distance] = find_closest_window_point(x,y,x_array,y_array, window, global_search, previous_location)
distance = 1e6;
location = previous_location;
array_length = length (x_array);

if (global_search == 1)
    
    %Search the whole array (usually at startup)
    for i =1:array_length
        d = (x-x_array(i))^2 + (y-y_array(i))^2;
        if d < distance
            distance = d;
            location = i;
        end
    end
    
else
    
    if (location + window) > array_length
        %We need to wrap from the end
        % loop one - end of array:
        for i = (location-window):array_length
            d = (x-x_array(i))^2 + (y-y_array(i))^2;
            if d < distance
                distance = d;
                location = i;
            end
        end
        % loop two - start of array:
        for i = 1:(location+window-array_length)
            d = (x-x_array(i))^2 + (y-y_array(i))^2;
            if d < distance
                distance = d;
                location = i;
            end
        end
        
    elseif (location-window) < 1
        %We need to wrap from the beginning
        % loop one - end of array:
        for i = (array_length+location-window):array_length
            d = (x-x_array(i))^2 + (y-y_array(i))^2;
            if d < distance
                distance = d;
                location = i;
            end
        end
        % loop two - start of array:
        for i = 1:(location+window)
            d = (x-x_array(i))^2 + (y-y_array(i))^2;
            if d < distance
                distance = d;
                location = i;
            end
        end
        
    else
        %no need to wrap
        for i = (location-window):(location+window)
            d = (x-x_array(i))^2 + (y-y_array(i))^2;
            if d < distance
                distance = d;
                location = i;
            end
        end
    end
    
end
distance = sqrt(distance);
end

== matlab function Smart_City_QCar2_self_driving_stack/Speed & Steering Commander/Traffic Zone 1/MATLAB Function2 ==
  data: Previous_State input; Speed_In input; Speed_Multi input; In_Zone input; Traffic_State output; Speed_Out output; Traffic_Light input
function [Traffic_State, Speed_Out]  = Traffic_Controller (Previous_State, Speed_In, Speed_Multi, In_Zone, Traffic_Light)
%#codegen
Traffic_State = Previous_State;
Speed_Out = Speed_In;

switch Traffic_State
    % Case 1 - Normal - either not in zone or green light, Case 2 - red
    % light and in zone
    
    case 1
        % Green light or not in zone
        Speed_Out = Speed_In;
        if (Traffic_Light == 0) && (In_Zone == 1)
            % Caught in the traffic controller's web!
            Traffic_State = 2;
        end
        
    case 2
        % Red light state
        Speed_Out = Speed_In * Speed_Multi;
        
        if (Traffic_Light == 1)
            % Green Light
            Traffic_State = 1;
        end
        
end
end

== matlab function Smart_City_QCar2_self_driving_stack/Speed & Steering Commander/MATLAB Function2 ==
  data: Previous_State input; Signs_In input; Stop_Sign input; Slow_Sign input; Sign_Time input; Sign_State output; Speed_Multiplier output; Signs_Out output; Step_size input; Previous_Timer input; Timer output
function [Sign_State, Speed_Multiplier, Signs_Out, Timer]  = NN_Decipher (Previous_State, Signs_In, Stop_Sign, Slow_Sign, Sign_Time, Step_size,Previous_Timer)
%#codegen
Sign_State = Previous_State;
Timer = Previous_Timer + Step_size;
Speed_Multiplier = 1;
Signs_Out = [0 Signs_In(2) Slow_Sign Stop_Sign Signs_In(5)];

switch Sign_State
    % Case 1 - No Sign, Case 2 - Stop Sign, Case 3 - Slow Sign
    
    case 1
        % No Signs Found
        Speed_Multiplier = 1;
        if (Timer > Sign_Time)
            % Stay in the No Sign state for a while each time
            if (Stop_Sign == 1)
                Sign_State = 2;
                Timer = 0;
            elseif  (Slow_Sign == 1)
                Sign_State = 3;
                Timer = 0;
            end
        end
        
    case 2
        % Stop Sign State
        Speed_Multiplier = 0;
        %         Signs_Out = [0 Signs_In(2) Slow_Sign 1 Signs_In(5)];
        Signs_Out = [0 0 0 1 0];
        if (Timer > Sign_Time)
            % Goto Normal State
            Sign_State = 1;
            Timer = 0;
        end
        
    case 3
        % Slow Sign State
        Speed_Multiplier = 0.5;
        %         Signs_Out = [0 Signs_In(2) 1 Stop_Sign Signs_In(5)];
        Signs_Out = [0 0 1 0 0];
        if (Timer > Sign_Time)
            % Goto Normal State
            Sign_State = 1;
            Timer = 0;
        end
        
end
end

== matlab function Smart_City_QCar2_self_driving_stack/Infrastructure/Find Closest Car/MATLAB Function ==
  data: x_car input; distance output; y_car input; x_vector input; y_vector input; car_index input; heading input; proximity_radius input; proximity_scan_window input; max_distance input; distance_vector output; heading_vector output
function [distance, distance_vector, heading_vector] = proximity_sensor (x_car, y_car, x_vector, y_vector, car_index, heading, proximity_radius, proximity_scan_window, max_distance)
distance = max_distance;
distance_vector = max_distance + 0*x_vector;
heading_vector = 2*pi +  0*x_vector;

for i = 1:length (x_vector)
    if (i ~= car_index)
        distance_vector(i) = sqrt ((x_car - x_vector(i))^2 + (y_car - y_vector(i))^2);
        heading_vector(i) = atan2( (y_vector(i) - y_car), (x_vector(i) - x_car)) - heading;
        if (heading_vector(i) > pi)
            heading_vector(i) = heading_vector(i) - 2*pi;
        elseif (heading_vector(i) < -pi)
            heading_vector(i) = heading_vector(i) + 2*pi;
        end
        if ((distance_vector(i) < distance) && (abs (heading_vector(i)) <= proximity_scan_window))
            distance =  distance_vector(i);
        end
       
    end
end
